simulink model "KTB1_SMAH"  (R2020a)
settings: Solver=ode45  StartTime=0.0  StopTime=120  RelTol=1e-3
values from neighbouring files (symbols this model uses):
  max_X = 5100    [SAP.m]
  max_XX = 2    [SAP.m]
  max_XXX = 0.05    [SAP.m]
  max_XXXX = 1050    [SAP.m]
  max_XXXXX = 15    [SAP.m]
  min_X = 0    [SAP.m]
  min_XX = 0    [SAP.m]
  min_XXX = 0    [SAP.m]
  min_XXXX = 0    [SAP.m]
  min_XXXXX = 0    [SAP.m]
  noiseseed = use2ndFcn    (= 1)    [SAP.m]
  noiseseed_X = use2ndFcn_X    (= 1)    [SAP.m]
  noiseseed_XX = use2ndFcn_XX    (= 1)    [SAP.m]
  noiseseed_XXX = use2ndFcn_XXX    (= 1)    [SAP.m]
  noiseseed_XXXX = use2ndFcn_XXXX    (= 1)    [SAP.m]
  noiseseed_XXXXX = use2ndFcn_XXXXX    (= 1)    [SAP.m]
  std = 0.025    [SAP.m]
  std_X = 0.025    [SAP.m]
  std_XX = 0.025    [SAP.m]
  std_XXX = 0.025    [SAP.m]
  std_XXXX = 0.025    [SAP.m]
  std_XXXXX = 0.025    [SAP.m]
  T_2 = T90_2/(24*60)/3.89    (= 0.000892602113682)    [SAP.m]
  T_8 = T90_8/(24*60)/11.7724    (= 0.00117978397683)    [SAP.m]
  T_X_2 = T90_X_2/(24*60)/3.89    (= 0.000892602113682)    [SAP.m]
  T_X_8 = T90_X_8/(24*60)/11.7724    (= 0.00117978397683)    [SAP.m]
  T_XX_2 = T90_XX_2/(24*60)/3.89    (= 0.000892602113682)    [SAP.m]
  T_XX_8 = T90_XX_8/(24*60)/11.7724    (= 0.00117978397683)    [SAP.m]
  T_XXX_2 = T90_XXX_2/(24*60)/3.89    (= 0.000892602113682)    [SAP.m]
  T_XXXX_2 = T90_XXXX_2/(24*60)/3.89    (= 0.000892602113682)    [SAP.m]
  T_XXXXX_2 = T90_XXXXX_2/(24*60)/3.89    (= 0.000892602113682)    [SAP.m]
  use2ndFcn = 1    [SAP.m]
  use2ndFcn_X = 1    [SAP.m]
  use2ndFcn_XX = 1    [SAP.m]
  use2ndFcn_XXX = 1    [SAP.m]
  use2ndFcn_XXXX = 1    [SAP.m]
  use2ndFcn_XXXXX = 1    [SAP.m]
  useideal = 1    [SAP.m]
  useideal_X = 1    [SAP.m]
  useideal_XX = 1    [SAP.m]
  useideal_XXX = 1    [SAP.m]
  useideal_XXXX = 1    [SAP.m]
  useideal_XXXXX = 1    [SAP.m]
  useidealac = 1    [SAP.m]
  useidealac_X = 1    [SAP.m]
  useidealac_XX = 1    [SAP.m]
  useidealac_XXX = 1    [SAP.m]
  useidealac_XXXX = 1    [SAP.m]
  useidealac_XXXXX = 1    [SAP.m]
  usenoise = 0    [SAP.m]
  usenoise_X = 0    [SAP.m]
  usenoise_XX = 0    [SAP.m]
  usenoise_XXX = 0    [SAP.m]
  usenoise_XXXX = 0    [SAP.m]
  usenoise_XXXXX = 0    [SAP.m]
libraries: simulink x6
(part 1 of 2)
settings Model: Creator=s182032  LastModifiedBy=morebo
settings DataIOCC: ReturnWorkspaceOutputs=off
settings DebuggingCC: MaxConsecutiveZCsMsg=none  ArithmeticOperatorsInVariantConditions=warning
settings SFSimCC: SimUseLocalCustomCode=off  CustomCodeUndefinedFunction=UseInterfaceOnly
settings RTWCC: RTWUseLocalCustomCode=off

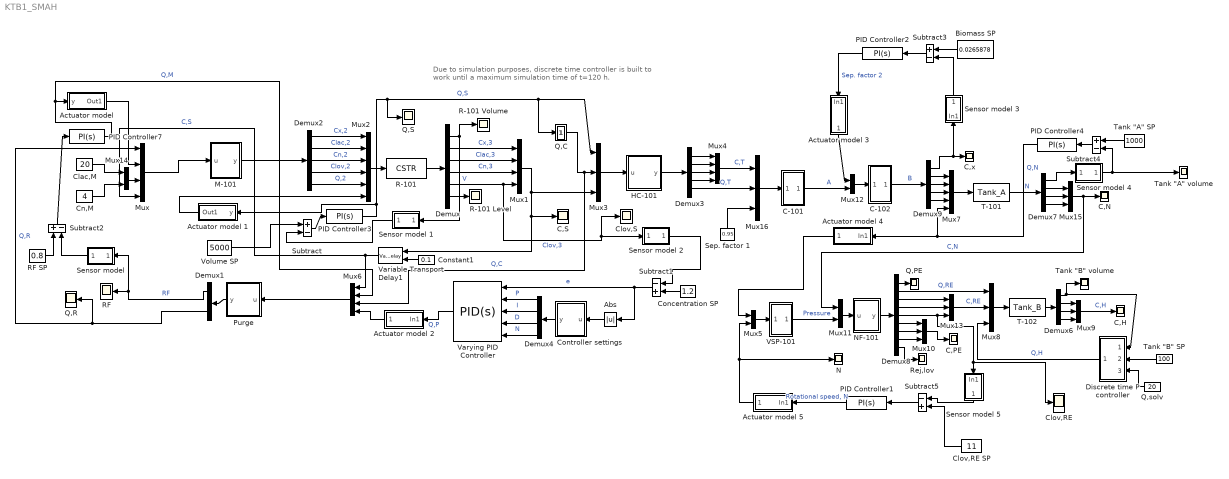
== system KTB1_SMAH ==
  note: Due to simulation purposes, discrete time controller is built to work until a maximum simulation time of t=120 h.
  Abs : Abs
  Actuator model : Subsystem
  Actuator model 1 : Subsystem
  Actuator model 2 : Subsystem
  Actuator model 3 : Subsystem
  Actuator model 4 : Subsystem
  Actuator model 5 : Subsystem
  Biomass SP : Constant  Value=0.0265878
  C,H : Scope
  C,N : Scope
  C,PE : Scope
  C,S : Scope
  C,x : Scope
  C-101 : MATLAB Function  TreatAsAtomicUnit=on
  C-102 : MATLAB Function  TreatAsAtomicUnit=on
  Clac,M : Constant  Value=20
  Clov,RE : Scope
  Clov,RE SP : Constant  Value=11
  Clov,S : Scope
  Cn,M : Constant  Value=4
  Concentration SP : Constant  Value=1.2
  Constant1 : Constant  Value=0.1
  Controller settings : MATLAB Function  TreatAsAtomicUnit=on
  Demux : Demux  Outputs=6
  Demux1 : Demux  Outputs=2
  Demux2 : Demux  Outputs=5
  Demux3 : Demux  Outputs=5
  Demux4 : Demux
  Demux6 : Demux
  Demux7 : Demux
  Demux8 : Demux  Outputs=9
  Demux9 : Demux  Outputs=5
  Discrete time P controller : Subsystem
  HC-101 : MATLAB Function  TreatAsAtomicUnit=on
  M-101 : MATLAB Function  TreatAsAtomicUnit=on
  Mux{,1,4,6} (4 alike) : Mux
  Mux{3,8..10,13,15..16} (7 alike) : Mux  Inputs=3
  Mux{5,11..12,14} (4 alike) : Mux  Inputs=2
  Mux2 : Mux  Inputs=6
  Mux7 : Mux  Inputs=5
  N : Scope
  NF-101 : MATLAB Function  TreatAsAtomicUnit=on
  PID Controller1 : simulink/Continuous/PID Controller  Controller=PI  Form=Parallel  TimeDomain=Continuous-time  UseExternalTs=off  SampleTime=-1  IntegratorMethod=Forward Euler  FilterMethod=Forward Euler  ControllerParametersSource=internal  P=0.234567821807165  I=0.999999996666666*0.234567821807165  D=0  UseFilter=on  N=100  TunerSelectOption=Transfer Function Based (PID Tuner App)  InitialConditionSource=internal  InitialConditionForIntegrator=3000  InitialConditionForFilter=0  DifferentiatorICPrevScaledInput=0  ExternalReset=none  TrackingMode=off  Kt=1  LimitOutput=on  UpperSaturationLimit=inf  LowerSaturationLimit=0  LinearizeAsGain=on  AntiWindupMode=clamping  Kb=1  POutMin=[]  POutMax=[]  IOutMin=[]  IOutMax=[]  DOutMin=[]  DOutMax=[]  NOutMin=[]  NOutMax=[]  SumOutMin=[]  SumOutMax=[]  SaturationOutMin=[]  SaturationOutMax=[]  PParamMin=[]  PParamMax=[]  IParamMin=[]  IParamMax=[]  DParamMin=[]  DParamMax=[]  NParamMin=[]  NParamMax=[]  KbParamMin=[]  KbParamMax=[]  KtParamMin=[]  KtParamMax=[]  KbOutMin=[]  KbOutMax=[]  KtOutMin=[]  KtOutMax=[]  IntegratorOutMin=[]  IntegratorOutMax=[]  FilterOutMin=[]  FilterOutMax=[]  SumI1OutMin=[]  SumI1OutMax=[]  SumI2OutMin=[]  SumI2OutMax=[]  SumI3OutMin=[]  SumI3OutMax=[]  SumI4OutMin=[]  SumI4OutMax=[]  SumDOutMin=[]  SumDOutMax=[]  DifferentiatorOutMin=[]  DifferentiatorOutMax=[]  FilterDiffOutCoefMin=[]  FilterDiffOutCoefMax=[]  ReciprocalOutMin=[]  ReciprocalOutMax=[]  SumDenOutMin=[]  SumDenOutMax=[]  SumNumOutMin=[]  SumNumOutMax=[]  DivideOutMin=[]  DivideOutMax=[]  UdiffTsProdOutMin=[]  UdiffTsProdOutMax=[]  NTsProdOutMin=[]  NTsProdOutMax=[]  UintegralTsProdOutMin=[]  UintegralTsProdOutMax=[]  UngainTsProdOutMin=[]  UngainTsProdOutMax=[]  IntegratorContinuousStateAttributes=''  IntegratorStateMustResolveToSignalObject=off  IntegratorRTWStateStorageClass=Auto  FilterContinuousStateAttributes=''  FilterStateMustResolveToSignalObject=off  FilterRTWStateStorageClass=Auto  ParallelPVariant=InternalParameters  IdealPVariant=Disabled  IVariant=InternalParameters  DVariant=Disabled  IntegratorVariant=Continuous  SatVariant=Enabled  AWVariant=ContClampingParallel  PCopyVariant=Disabled  TRVariant=Disabled  FdbkBlocksVariant=Forward  IdealPFdbkVariant=Disabled  SatFdbkVariant=Disabled  DerivativeFilterVariant=Disabled  NVariant=Disabled  NCopyVariant=Disabled_SignalSpec  FilterICVariant=Disabled  IntegratorICVariant=InternalICs  ExternalResetVariant=Disabled  TRSumVariant=Passthrough  SumFdbkVariant=Disabled  SumVariant=Sum_PI  TsampFilterVariant=InternalTs  TsampNgainVariant=Passthrough  TsampIntegralVariant=Passthrough
  PID Controller2 : simulink/Continuous/PID Controller  Controller=PI  Form=Parallel  TimeDomain=Continuous-time  UseExternalTs=off  SampleTime=-1  IntegratorMethod=Forward Euler  FilterMethod=Forward Euler  ControllerParametersSource=internal  P=-0.000476190628986061  I=9.99999996666667*(-0.000476190628986061)  D=0  UseFilter=on  N=100  TunerSelectOption=Transfer Function Based (PID Tuner App)  InitialConditionSource=internal  InitialConditionForIntegrator=0.95  InitialConditionForFilter=0  DifferentiatorICPrevScaledInput=0  ExternalReset=none  TrackingMode=off  Kt=1  LimitOutput=on  UpperSaturationLimit=0.98  LowerSaturationLimit=0  LinearizeAsGain=on  AntiWindupMode=clamping  Kb=1  POutMin=[]  POutMax=[]  IOutMin=[]  IOutMax=[]  DOutMin=[]  DOutMax=[]  NOutMin=[]  NOutMax=[]  SumOutMin=[]  SumOutMax=[]  SaturationOutMin=[]  SaturationOutMax=[]  PParamMin=[]  PParamMax=[]  IParamMin=[]  IParamMax=[]  DParamMin=[]  DParamMax=[]  NParamMin=[]  NParamMax=[]  KbParamMin=[]  KbParamMax=[]  KtParamMin=[]  KtParamMax=[]  KbOutMin=[]  KbOutMax=[]  KtOutMin=[]  KtOutMax=[]  IntegratorOutMin=[]  IntegratorOutMax=[]  FilterOutMin=[]  FilterOutMax=[]  SumI1OutMin=[]  SumI1OutMax=[]  SumI2OutMin=[]  SumI2OutMax=[]  SumI3OutMin=[]  SumI3OutMax=[]  SumI4OutMin=[]  SumI4OutMax=[]  SumDOutMin=[]  SumDOutMax=[]  DifferentiatorOutMin=[]  DifferentiatorOutMax=[]  FilterDiffOutCoefMin=[]  FilterDiffOutCoefMax=[]  ReciprocalOutMin=[]  ReciprocalOutMax=[]  SumDenOutMin=[]  SumDenOutMax=[]  SumNumOutMin=[]  SumNumOutMax=[]  DivideOutMin=[]  DivideOutMax=[]  UdiffTsProdOutMin=[]  UdiffTsProdOutMax=[]  NTsProdOutMin=[]  NTsProdOutMax=[]  UintegralTsProdOutMin=[]  UintegralTsProdOutMax=[]  UngainTsProdOutMin=[]  UngainTsProdOutMax=[]  IntegratorContinuousStateAttributes=''  IntegratorStateMustResolveToSignalObject=off  IntegratorRTWStateStorageClass=Auto  FilterContinuousStateAttributes=''  FilterStateMustResolveToSignalObject=off  FilterRTWStateStorageClass=Auto  ParallelPVariant=InternalParameters  IdealPVariant=Disabled  IVariant=InternalParameters  DVariant=Disabled  IntegratorVariant=Continuous  SatVariant=Enabled  AWVariant=ContClampingParallel  PCopyVariant=Disabled  TRVariant=Disabled  FdbkBlocksVariant=Forward  IdealPFdbkVariant=Disabled  SatFdbkVariant=Disabled  DerivativeFilterVariant=Disabled  NVariant=Disabled  NCopyVariant=Disabled_SignalSpec  FilterICVariant=Disabled  IntegratorICVariant=InternalICs  ExternalResetVariant=Disabled  TRSumVariant=Passthrough  SumFdbkVariant=Disabled  SumVariant=Sum_PI  TsampFilterVariant=InternalTs  TsampNgainVariant=Passthrough  TsampIntegralVariant=Passthrough
  PID Controller3 : simulink/Continuous/PID Controller  Controller=PI  Form=Parallel  TimeDomain=Continuous-time  UseExternalTs=off  SampleTime=-1  IntegratorMethod=Forward Euler  FilterMethod=Forward Euler  ControllerParametersSource=internal  P=-1/0.4/0.2  I=-1/0.4/0.2/4/0.2  D=0  UseFilter=on  N=100  TunerSelectOption=Transfer Function Based (PID Tuner App)  InitialConditionSource=internal  InitialConditionForIntegrator=64.0830509473650  InitialConditionForFilter=0  DifferentiatorICPrevScaledInput=0  ExternalReset=none  TrackingMode=off  Kt=1  LimitOutput=on  UpperSaturationLimit=inf  LowerSaturationLimit=0  LinearizeAsGain=on  AntiWindupMode=clamping  Kb=1  POutMin=[]  POutMax=[]  IOutMin=[]  IOutMax=[]  DOutMin=[]  DOutMax=[]  NOutMin=[]  NOutMax=[]  SumOutMin=[]  SumOutMax=[]  SaturationOutMin=[]  SaturationOutMax=[]  PParamMin=[]  PParamMax=[]  IParamMin=[]  IParamMax=[]  DParamMin=[]  DParamMax=[]  NParamMin=[]  NParamMax=[]  KbParamMin=[]  KbParamMax=[]  KtParamMin=[]  KtParamMax=[]  KbOutMin=[]  KbOutMax=[]  KtOutMin=[]  KtOutMax=[]  IntegratorOutMin=[]  IntegratorOutMax=[]  FilterOutMin=[]  FilterOutMax=[]  SumI1OutMin=[]  SumI1OutMax=[]  SumI2OutMin=[]  SumI2OutMax=[]  SumI3OutMin=[]  SumI3OutMax=[]  SumI4OutMin=[]  SumI4OutMax=[]  SumDOutMin=[]  SumDOutMax=[]  DifferentiatorOutMin=[]  DifferentiatorOutMax=[]  FilterDiffOutCoefMin=[]  FilterDiffOutCoefMax=[]  ReciprocalOutMin=[]  ReciprocalOutMax=[]  SumDenOutMin=[]  SumDenOutMax=[]  SumNumOutMin=[]  SumNumOutMax=[]  DivideOutMin=[]  DivideOutMax=[]  UdiffTsProdOutMin=[]  UdiffTsProdOutMax=[]  NTsProdOutMin=[]  NTsProdOutMax=[]  UintegralTsProdOutMin=[]  UintegralTsProdOutMax=[]  UngainTsProdOutMin=[]  UngainTsProdOutMax=[]  IntegratorContinuousStateAttributes=''  IntegratorStateMustResolveToSignalObject=off  IntegratorRTWStateStorageClass=Auto  FilterContinuousStateAttributes=''  FilterStateMustResolveToSignalObject=off  FilterRTWStateStorageClass=Auto  ParallelPVariant=InternalParameters  IdealPVariant=Disabled  IVariant=InternalParameters  DVariant=Disabled  IntegratorVariant=Continuous  SatVariant=Enabled  AWVariant=ContClampingParallel  PCopyVariant=Disabled  TRVariant=Disabled  FdbkBlocksVariant=Forward  IdealPFdbkVariant=Disabled  SatFdbkVariant=Disabled  DerivativeFilterVariant=Disabled  NVariant=Disabled  NCopyVariant=Disabled_SignalSpec  FilterICVariant=Disabled  IntegratorICVariant=InternalICs  ExternalResetVariant=Disabled  TRSumVariant=Passthrough  SumFdbkVariant=Disabled  SumVariant=Sum_PI  TsampFilterVariant=InternalTs  TsampNgainVariant=Passthrough  TsampIntegralVariant=Passthrough
  PID Controller4 : simulink/Continuous/PID Controller  Controller=PI  Form=Parallel  TimeDomain=Continuous-time  UseExternalTs=off  SampleTime=-1  IntegratorMethod=Forward Euler  FilterMethod=Forward Euler  ControllerParametersSource=internal  P=-1/140  I=-1/4/140/140  D=0  UseFilter=on  N=100  TunerSelectOption=Transfer Function Based (PID Tuner App)  InitialConditionSource=internal  InitialConditionForIntegrator=25.6332203789471  InitialConditionForFilter=0  DifferentiatorICPrevScaledInput=0  ExternalReset=none  TrackingMode=off  Kt=1  LimitOutput=on  UpperSaturationLimit=inf  LowerSaturationLimit=0  LinearizeAsGain=on  AntiWindupMode=clamping  Kb=1  POutMin=[]  POutMax=[]  IOutMin=[]  IOutMax=[]  DOutMin=[]  DOutMax=[]  NOutMin=[]  NOutMax=[]  SumOutMin=[]  SumOutMax=[]  SaturationOutMin=[]  SaturationOutMax=[]  PParamMin=[]  PParamMax=[]  IParamMin=[]  IParamMax=[]  DParamMin=[]  DParamMax=[]  NParamMin=[]  NParamMax=[]  KbParamMin=[]  KbParamMax=[]  KtParamMin=[]  KtParamMax=[]  KbOutMin=[]  KbOutMax=[]  KtOutMin=[]  KtOutMax=[]  IntegratorOutMin=[]  IntegratorOutMax=[]  FilterOutMin=[]  FilterOutMax=[]  SumI1OutMin=[]  SumI1OutMax=[]  SumI2OutMin=[]  SumI2OutMax=[]  SumI3OutMin=[]  SumI3OutMax=[]  SumI4OutMin=[]  SumI4OutMax=[]  SumDOutMin=[]  SumDOutMax=[]  DifferentiatorOutMin=[]  DifferentiatorOutMax=[]  FilterDiffOutCoefMin=[]  FilterDiffOutCoefMax=[]  ReciprocalOutMin=[]  ReciprocalOutMax=[]  SumDenOutMin=[]  SumDenOutMax=[]  SumNumOutMin=[]  SumNumOutMax=[]  DivideOutMin=[]  DivideOutMax=[]  UdiffTsProdOutMin=[]  UdiffTsProdOutMax=[]  NTsProdOutMin=[]  NTsProdOutMax=[]  UintegralTsProdOutMin=[]  UintegralTsProdOutMax=[]  UngainTsProdOutMin=[]  UngainTsProdOutMax=[]  IntegratorContinuousStateAttributes=''  IntegratorStateMustResolveToSignalObject=off  IntegratorRTWStateStorageClass=Auto  FilterContinuousStateAttributes=''  FilterStateMustResolveToSignalObject=off  FilterRTWStateStorageClass=Auto  ParallelPVariant=InternalParameters  IdealPVariant=Disabled  IVariant=InternalParameters  DVariant=Disabled  IntegratorVariant=Continuous  SatVariant=Enabled  AWVariant=ContClampingParallel  PCopyVariant=Disabled  TRVariant=Disabled  FdbkBlocksVariant=Forward  IdealPFdbkVariant=Disabled  SatFdbkVariant=Disabled  DerivativeFilterVariant=Disabled  NVariant=Disabled  NCopyVariant=Disabled_SignalSpec  FilterICVariant=Disabled  IntegratorICVariant=InternalICs  ExternalResetVariant=Disabled  TRSumVariant=Passthrough  SumFdbkVariant=Disabled  SumVariant=Sum_PI  TsampFilterVariant=InternalTs  TsampNgainVariant=Passthrough  TsampIntegralVariant=Passthrough
  PID Controller7 : simulink/Continuous/PID Controller  Controller=PI  Form=Parallel  TimeDomain=Continuous-time  UseExternalTs=off  SampleTime=-1  IntegratorMethod=Forward Euler  FilterMethod=Forward Euler  ControllerParametersSource=internal  P=4.68116891262785/100  I=30.3539293345611/100  D=0  UseFilter=on  N=100  TunerSelectOption=Transfer Function Based (PID Tuner App)  InitialConditionSource=internal  InitialConditionForIntegrator=35.6016949707568  InitialConditionForFilter=0  DifferentiatorICPrevScaledInput=0  ExternalReset=none  TrackingMode=off  Kt=1  LimitOutput=on  UpperSaturationLimit=inf  LowerSaturationLimit=0  LinearizeAsGain=on  AntiWindupMode=clamping  Kb=1  POutMin=[]  POutMax=[]  IOutMin=[]  IOutMax=[]  DOutMin=[]  DOutMax=[]  NOutMin=[]  NOutMax=[]  SumOutMin=[]  SumOutMax=[]  SaturationOutMin=[]  SaturationOutMax=[]  PParamMin=[]  PParamMax=[]  IParamMin=[]  IParamMax=[]  DParamMin=[]  DParamMax=[]  NParamMin=[]  NParamMax=[]  KbParamMin=[]  KbParamMax=[]  KtParamMin=[]  KtParamMax=[]  KbOutMin=[]  KbOutMax=[]  KtOutMin=[]  KtOutMax=[]  IntegratorOutMin=[]  IntegratorOutMax=[]  FilterOutMin=[]  FilterOutMax=[]  SumI1OutMin=[]  SumI1OutMax=[]  SumI2OutMin=[]  SumI2OutMax=[]  SumI3OutMin=[]  SumI3OutMax=[]  SumI4OutMin=[]  SumI4OutMax=[]  SumDOutMin=[]  SumDOutMax=[]  DifferentiatorOutMin=[]  DifferentiatorOutMax=[]  FilterDiffOutCoefMin=[]  FilterDiffOutCoefMax=[]  ReciprocalOutMin=[]  ReciprocalOutMax=[]  SumDenOutMin=[]  SumDenOutMax=[]  SumNumOutMin=[]  SumNumOutMax=[]  DivideOutMin=[]  DivideOutMax=[]  UdiffTsProdOutMin=[]  UdiffTsProdOutMax=[]  NTsProdOutMin=[]  NTsProdOutMax=[]  UintegralTsProdOutMin=[]  UintegralTsProdOutMax=[]  UngainTsProdOutMin=[]  UngainTsProdOutMax=[]  IntegratorContinuousStateAttributes=''  IntegratorStateMustResolveToSignalObject=off  IntegratorRTWStateStorageClass=Auto  FilterContinuousStateAttributes=''  FilterStateMustResolveToSignalObject=off  FilterRTWStateStorageClass=Auto  ParallelPVariant=InternalParameters  IdealPVariant=Disabled  IVariant=InternalParameters  DVariant=Disabled  IntegratorVariant=Continuous  SatVariant=Enabled  AWVariant=ContClampingParallel  PCopyVariant=Disabled  TRVariant=Disabled  FdbkBlocksVariant=Forward  IdealPFdbkVariant=Disabled  SatFdbkVariant=Disabled  DerivativeFilterVariant=Disabled  NVariant=Disabled  NCopyVariant=Disabled_SignalSpec  FilterICVariant=Disabled  IntegratorICVariant=InternalICs  ExternalResetVariant=Disabled  TRSumVariant=Passthrough  SumFdbkVariant=Disabled  SumVariant=Sum_PI  TsampFilterVariant=InternalTs  TsampNgainVariant=Passthrough  TsampIntegralVariant=Passthrough
  Purge : MATLAB Function  TreatAsAtomicUnit=on
  Q,C : Subsystem
  Q,PE : Scope
  Q,R : Scope
  Q,S : Scope
  Q,solv : Constant  Value=20
  R-101 : S-Function  FunctionName=CSTR  SFunctionDeploymentMode=off  EnableBusSupport=off
  R-101 Level : Scope
  R-101 Volume : Scope
  RF : Scope
  RF SP : Constant  Value=0.8
  Rej,lov : Scope
  Sensor model : Subsystem
  Sensor model 1 : Subsystem
  Sensor model 2 : Subsystem
  Sensor model 3 : Subsystem
  Sensor model 4 : Subsystem
  Sensor model 5 : Subsystem
  Sep. factor 1 : Constant  Value=0.95
  Subtract{,2..4} (4 alike) : Sum  Inputs=+-
  Subtract1 : Sum  Inputs=-+
  Subtract5 : Sum  Inputs=-+
  T-101 : S-Function  FunctionName=Tank_A  SFunctionDeploymentMode=off  EnableBusSupport=off
  T-102 : S-Function  FunctionName=Tank_B  SFunctionDeploymentMode=off  EnableBusSupport=off
  "Tank \"A\" SP" : Constant  Value=1000
  "Tank \"A\" volume" : Scope
  "Tank \"B\" SP" : Constant  Value=100
  "Tank \"B\" volume" : Scope
  VSP-101 : MATLAB Function  TreatAsAtomicUnit=on
  Variable Transport Delay1 : VariableTransportDelay  VariableDelayType=Variable transport delay  MaximumDelay=10  InitialOutput=[106.351163614666 14.8096563646109 2.51553709810012 1.20000000000003]  MaximumPoints=80000
  Varying PID Controller : simulink/Continuous/PID Controller  Controller=PID  Form=Parallel  TimeDomain=Continuous-time  UseExternalTs=off  SampleTime=-1  IntegratorMethod=Forward Euler  FilterMethod=Forward Euler  ControllerParametersSource=external  P=1  I=1  D=0  UseFilter=on  N=100  TunerSelectOption=Transfer Function Based (PID Tuner App)  InitialConditionSource=internal  InitialConditionForIntegrator=9.96847459181301  InitialConditionForFilter=0  DifferentiatorICPrevScaledInput=0  ExternalReset=none  TrackingMode=off  Kt=1  LimitOutput=on  UpperSaturationLimit=inf  LowerSaturationLimit=0  LinearizeAsGain=on  AntiWindupMode=none  Kb=1  POutMin=[]  POutMax=[]  IOutMin=[]  IOutMax=[]  DOutMin=[]  DOutMax=[]  NOutMin=[]  NOutMax=[]  SumOutMin=[]  SumOutMax=[]  SaturationOutMin=[]  SaturationOutMax=[]  PParamMin=[]  PParamMax=[]  IParamMin=[]  IParamMax=[]  DParamMin=[]  DParamMax=[]  NParamMin=[]  NParamMax=[]  KbParamMin=[]  KbParamMax=[]  KtParamMin=[]  KtParamMax=[]  KbOutMin=[]  KbOutMax=[]  KtOutMin=[]  KtOutMax=[]  IntegratorOutMin=[]  IntegratorOutMax=[]  FilterOutMin=[]  FilterOutMax=[]  SumI1OutMin=[]  SumI1OutMax=[]  SumI2OutMin=[]  SumI2OutMax=[]  SumI3OutMin=[]  SumI3OutMax=[]  SumI4OutMin=[]  SumI4OutMax=[]  SumDOutMin=[]  SumDOutMax=[]  DifferentiatorOutMin=[]  DifferentiatorOutMax=[]  FilterDiffOutCoefMin=[]  FilterDiffOutCoefMax=[]  ReciprocalOutMin=[]  ReciprocalOutMax=[]  SumDenOutMin=[]  SumDenOutMax=[]  SumNumOutMin=[]  SumNumOutMax=[]  DivideOutMin=[]  DivideOutMax=[]  UdiffTsProdOutMin=[]  UdiffTsProdOutMax=[]  NTsProdOutMin=[]  NTsProdOutMax=[]  UintegralTsProdOutMin=[]  UintegralTsProdOutMax=[]  UngainTsProdOutMin=[]  UngainTsProdOutMax=[]  IntegratorContinuousStateAttributes=''  IntegratorStateMustResolveToSignalObject=off  IntegratorRTWStateStorageClass=Auto  FilterContinuousStateAttributes=''  FilterStateMustResolveToSignalObject=off  FilterRTWStateStorageClass=Auto  ParallelPVariant=ExternalParameters  IdealPVariant=Disabled  IVariant=ExternalParameters  DVariant=ExternalParameters  IntegratorVariant=Continuous  SatVariant=Enabled  AWVariant=Passthrough  PCopyVariant=Disabled  TRVariant=Disabled  FdbkBlocksVariant=Forward  IdealPFdbkVariant=Disabled  SatFdbkVariant=Disabled  DerivativeFilterVariant=ContFilter  NVariant=ExternalParameters  NCopyVariant=Disabled  FilterICVariant=InternalICsFilter  IntegratorICVariant=InternalICs  ExternalResetVariant=Disabled  TRSumVariant=Passthrough  SumFdbkVariant=Disabled  SumVariant=Sum_PID  TsampFilterVariant=InternalTs  TsampNgainVariant=Passthrough  TsampIntegralVariant=Passthrough
  Volume SP : Constant  Value=5000
  wires:
  Concentration SP/1 -> Subtract1/2
  Demux4/1 -> Varying PID Controller/2  "P"
  Subtract1/1 -> Abs/1, Varying PID Controller/1  "e"
  Demux4/2 -> Varying PID Controller/3  "I"
  PID Controller7/1 -> Actuator model/1(y), Mux6/2  "Q,M"
  Varying PID Controller/1 -> Actuator model 2/1(In1)  "Q,P"
  Demux2/5 -> Mux2/5  "Q,2"
  Mux6/1 -> Purge/1(u)
  Demux2/4 -> Mux2/4  "Clov,2"
  Demux3/1 -> Mux4/1
  Purge/1(y) -> Demux1/1
  Demux2/3 -> Mux2/3  "Cn,2"
  Demux3/2 -> Mux4/2
  Demux3/3 -> Mux4/3
  HC-101/1(y) -> Demux3/1
  Mux3/1 -> HC-101/1(u)
  Demux2/2 -> Mux2/2  "Clac,2"
  PID Controller3/1 -> Actuator model 1/1(y), Q,C/1(Qs), Mux3/1, Q,S/1  "Q,S"
  Demux/1 -> Sensor model 1/1(In1), R-101 Volume/1  "V"
  Demux/2 -> Mux1/1  "Cx,3"
  Demux/3 -> Mux1/2  "Clac,3"
  Mux/1 -> M-101/1(u)
  Mux2/1 -> R-101/1
  Demux2/1 -> Mux2/1  "Cx,2"
  Variable Transport Delay1/1 -> Mux/4, Mux6/1  "C,S"
  R-101/1 -> Demux/1
  Mux1/1 -> C,S/1, Variable Transport Delay1/1, Mux3/3
  Constant1/1 -> Variable Transport Delay1/2
  M-101/1(y) -> Demux2/1
  Demux/4 -> Mux1/3  "Cn,3"
  Demux/5 -> Clov,S/1, Sensor model 2/1(In1), Mux1/4  "Clov,3"
  Subtract/1 -> PID Controller3/1
  Demux3/4 -> Mux4/4
  Cn,M/1 -> Mux14/2
  Demux/6 -> R-101 Level/1
  Mux14/1 -> Mux/3
  Demux1/2 -> Mux/1, Q,R/1  "Q,R"
  Volume SP/1 -> Subtract/1
  Demux1/1 -> Sensor model/1(In1), RF/1  "RF"
  Clac,M/1 -> Mux14/1
  Abs/1 -> Controller settings/1(u)
  Controller settings/1(y) -> Demux4/1
  Demux4/3 -> Varying PID Controller/4  "D"
  Demux4/4 -> Varying PID Controller/5  "N"
  RF SP/1 -> Subtract2/1
  Subtract2/1 -> PID Controller7/1
  Q,C/1(Qc) -> Mux6/3, Mux3/2  "Q,C"
  Demux6/1 -> Discrete time P controller/1(In1), "Tank \"B\" volume"/1
  Discrete time P controller/1(Q,H) -> Mux8/3  "Q,H"
  Q,solv/1 -> Discrete time P controller/3(In3)
  "Tank \"B\" SP"/1 -> Discrete time P controller/2(In2)
  Demux9/4 -> Mux7/3
  Clov,RE SP/1 -> Subtract5/2
  Subtract3/1 -> PID Controller2/1
  C-102/1(y) -> Demux9/1  "B"
  Demux8/9 -> Rej,lov/1
  PID Controller1/1 -> Actuator model 5/1(In1)  "Rotational speed, N"
  Demux9/1 -> Sensor model 3/1(In1), C,x/1
  Demux7/3 -> Mux15/2
  Demux8/8 -> Mux10/3
  Demux9/2 -> Mux7/1
  Mux5/1 -> VSP-101/1(u)
  VSP-101/1(y) -> Mux11/2  "Pressure"
  Demux6/2 -> Mux9/1
  T-102/1 -> Demux6/1
  Demux9/5 -> Mux7/4
  Demux8/2 -> Mux8/1  "Q,RE"
  Demux6/3 -> Mux9/2
  Mux15/1 -> Mux11/1, C,N/1  "C,N"
  Mux7/1 -> T-101/1
  Demux9/3 -> Mux7/2
  Demux8/3 -> Mux13/1
  Mux8/1 -> T-102/1
  Mux10/1 -> C,PE/1
  Demux8/4 -> Mux13/2
  Subtract4/1 -> PID Controller4/1
  PID Controller4/1 -> Actuator model 4/1(In1), Mux7/5  "Q,N"
  Subtract5/1 -> PID Controller1/1
  Demux8/7 -> Mux10/2
  Demux6/4 -> Mux9/3
  Mux16/1 -> C-101/1(u)
  Sep. factor 1/1 -> Mux16/3
  Mux11/1 -> NF-101/1(u)
  NF-101/1(y) -> Demux8/1
  "Tank \"A\" SP"/1 -> Subtract4/1
  Mux9/1 -> C,H/1  "C,H"
  T-101/1 -> Demux7/1  "N"
  Mux13/1 -> Mux8/2  "C,RE"
  Mux12/1 -> C-102/1(u)
  Biomass SP/1 -> Subtract3/1
  Demux8/6 -> Mux10/1
  Demux7/4 -> Mux15/3
  Demux8/1 -> Q,PE/1
  C-101/1(y) -> Mux12/2  "A"
  Demux7/2 -> Mux15/1
  PID Controller2/1 -> Actuator model 3/1(In1)  "Sep. factor 2"
  Mux4/1 -> Mux16/1  "C,T"
  Demux3/5 -> Mux16/2  "Q,T"
  Sensor model 2/1(Out1) -> Subtract1/1
  Actuator model 2/1(Out1) -> Mux6/4
  Sensor model/1(Out1) -> Subtract2/2
  Actuator model/1(Out1) -> Mux/2
  Sensor model 1/1(Out1) -> Subtract/2
  Actuator model 1/1(Out1) -> Mux2/6
  Sensor model 3/1(Out1) -> Subtract3/2
  Actuator model 3/1(Out1) -> Mux12/1
  Demux7/1 -> Sensor model 4/1(In1)
  Demux8/5 -> Clov,RE/1, Sensor model 5/1(In1), Mux13/3
  Sensor model 4/1(Out1) -> Subtract4/2, "Tank \"A\" volume"/1
  Actuator model 4/1(Out1) -> Mux5/1
  Sensor model 5/1(Out1) -> Subtract5/1
  Actuator model 5/1(Out1) -> Mux5/2, N/1

== system KTB1_SMAH/Actuator model ==
  y : Inport
  Constant2 : Constant  Value=useidealac
  Switch1 : Switch  Threshold=0.5
  actuator : TransferFcn  Denominator=[ T_2*T_2, 2*T_2, 1]
  Out1 : Outport
  wires:
  Constant2/1 -> Switch1/2
  y/1 -> Switch1/1, actuator/1
  actuator/1 -> Switch1/3
  Switch1/1 -> Out1/1

== system KTB1_SMAH/Actuator model 1 ==
  y : Inport
  Constant2 : Constant  Value=useidealac_X
  Switch1 : Switch  Threshold=0.5
  X_actuator : TransferFcn  Denominator=[ T_X_2*T_X_2, 2*T_X_2, 1]
  Out1 : Outport
  wires:
  Constant2/1 -> Switch1/2
  y/1 -> Switch1/1, X_actuator/1
  X_actuator/1 -> Switch1/3
  Switch1/1 -> Out1/1

== system KTB1_SMAH/Actuator model 2 ==
  In1 : Inport
  Constant2 : Constant  Value=useidealac_XX
  Switch1 : Switch  Threshold=0.5
  XX_actuator : TransferFcn  Denominator=[ T_XX_2*T_XX_2, 2*T_XX_2, 1]
  Out1 : Outport
  wires:
  Constant2/1 -> Switch1/2
  In1/1 -> Switch1/1, XX_actuator/1
  XX_actuator/1 -> Switch1/3
  Switch1/1 -> Out1/1

== system KTB1_SMAH/Actuator model 3 ==
  In1 : Inport
  Constant2 : Constant  Value=useidealac_XXX
  Switch1 : Switch  Threshold=0.5
  XXX_actuator : TransferFcn  Denominator=[ T_XXX_2*T_XXX_2, 2*T_XXX_2, 1]
  Out1 : Outport
  wires:
  Constant2/1 -> Switch1/2
  In1/1 -> Switch1/1, XXX_actuator/1
  XXX_actuator/1 -> Switch1/3
  Switch1/1 -> Out1/1

== system KTB1_SMAH/Actuator model 4 ==
  In1 : Inport
  Constant2 : Constant  Value=useidealac_XXXX
  Switch1 : Switch  Threshold=0.5
  XXXX_actuator : TransferFcn  Denominator=[ T_XXXX_2*T_XXXX_2, 2*T_XXXX_2, 1]
  Out1 : Outport
  wires:
  Constant2/1 -> Switch1/2
  In1/1 -> Switch1/1, XXXX_actuator/1
  XXXX_actuator/1 -> Switch1/3
  Switch1/1 -> Out1/1

== system KTB1_SMAH/Actuator model 5 ==
  In1 : Inport
  Constant2 : Constant  Value=useidealac_XXXXX
  Switch1 : Switch  Threshold=0.5
  XXXX_actuator : TransferFcn  Denominator=[ T_XXXXX_2*T_XXXXX_2, 2*T_XXXXX_2, 1]
  Out1 : Outport
  wires:
  Constant2/1 -> Switch1/2
  In1/1 -> Switch1/1, XXXX_actuator/1
  XXXX_actuator/1 -> Switch1/3
  Switch1/1 -> Out1/1

== system KTB1_SMAH/Discrete time P controller ==
  In1 : Inport
  In2 : Inport  Port=2
  In3 : Inport  Port=3
  1 : Subsystem
  10 : Subsystem
  2 : Subsystem
  3 : Subsystem
  4 : Subsystem
  5 : Subsystem
  6 : Subsystem
  7 : Subsystem
  8 : Subsystem
  9 : Subsystem
  Sum1 : Sum  Inputs=++++++++++
  Q,H : Outport  VectorParamsAs1DForOutWhenUnconnected=off
  wires:
  In3/1 -> 3/3(In3), 4/3(In3), 6/3(In3), 7/3(In3), 8/3(In3), 10/3(In3), 9/3(In3), 5/3(In3), 2/3(In3), 1/1(In1)
  In2/1 -> 2/2(In2), 3/2(In2), 4/2(In2), 5/2(In2), 6/2(In2), 8/2(In2), 10/2(In2), 9/2(In2), 7/2(In2)
  7/1(Out1) -> Sum1/7
  3/1(Out1) -> Sum1/3
  4/1(Out1) -> Sum1/4
  2/1(Out1) -> Sum1/2
  6/1(Out1) -> Sum1/6
  8/1(Out1) -> Sum1/8
  10/1(Out1) -> Sum1/10
  9/1(Out1) -> Sum1/9
  5/1(Out1) -> Sum1/5
  Sum1/1 -> Q,H/1  "Q,H"
  1/1(Out1) -> Sum1/1
  In1/1 -> 4/1(In1), 5/1(In1), 6/1(In1), 7/1(In1), 8/1(In1), 10/1(In1), 9/1(In1), 3/1(In1), 2/1(In1)

== system KTB1_SMAH/Q,C ==
  Qs : Inport
  Product1 : Product
  Q,C/Q,S : Constant  Value=0.6
  Qc : Outport  VectorParamsAs1DForOutWhenUnconnected=off
  wires:
  Product1/1 -> Qc/1  "Qc"
  Q,C/Q,S/1 -> Product1/1
  Qs/1 -> Product1/2

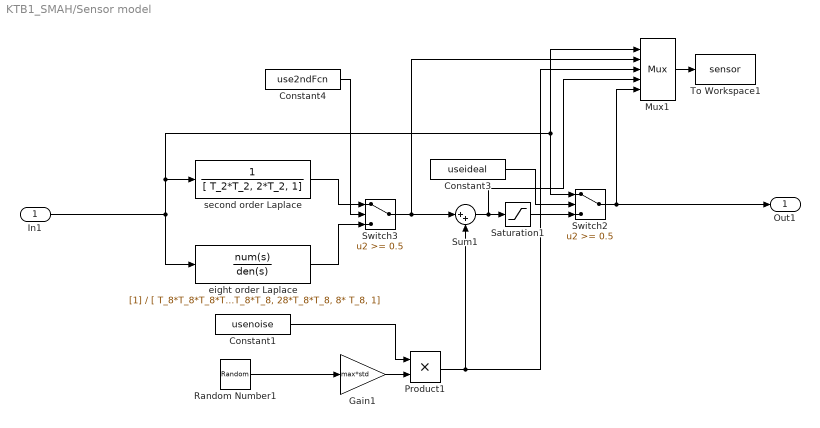
== system KTB1_SMAH/Sensor model ==
  In1 : Inport
  Constant1 : Constant  Value=usenoise
  Constant3 : Constant  Value=useideal
  Constant4 : Constant  Value=use2ndFcn
  Gain1 : Gain  Gain=max*std  SaturateOnIntegerOverflow=on  OutDataTypeStr=Inherit: Same as input  ParamDataTypeStr=Inherit: Same as input
  Mux1 : Mux  Inputs=5
  Product1 : Product  InputSameDT=on  SaturateOnIntegerOverflow=on  OutDataTypeStr=Inherit: Same as first input
  Random Number1 : RandomNumber  Seed=noiseseed  SampleTime=1/2
  Saturation1 : Saturate  UpperLimit=max  LowerLimit=min
  Sum1 : Sum  Inputs=|++  InputSameDT=on  SaturateOnIntegerOverflow=on  OutDataTypeStr=Inherit: Same as first input
  Switch2 : Switch  Threshold=0.5
  Switch3 : Switch  Threshold=0.5
  To Workspace1 : ToWorkspace  VariableName=sensor  SampleTime=-1
  eight order Laplace : TransferFcn  Denominator=[ T_8*T_8*T_8*T_8*T_8*T_8*T_8*T_8, 8*T_8*T_8*T_8*T_8*T_8*T_8*T_8, 28*T_8*T_8*T_8*T_8*T_8*T_8, 56*T_8*T_8*T_8*T_8*T_8, 70*T_8*T_8*T_8*T_8, 56*T_8*T_8*T_8, 28*T_8*T_8, 8* T_8, 1]
  second order Laplace : TransferFcn  Denominator=[ T_2*T_2, 2*T_2, 1]
  Out1 : Outport
  wires:
  Saturation1/1 -> Switch2/3
  In1/1 -> second order Laplace/1, Mux1/1, Switch2/1, eight order Laplace/1
  Constant1/1 -> Product1/1
  eight order Laplace/1 -> Switch3/3
  Constant4/1 -> Switch3/2
  Gain1/1 -> Product1/2
  Product1/1 -> Mux1/3, Sum1/2
  Switch2/1 -> Mux1/5, Out1/1
  Constant3/1 -> Switch2/2
  second order Laplace/1 -> Switch3/1
  Random Number1/1 -> Gain1/1
  Mux1/1 -> To Workspace1/1
  Sum1/1 -> Mux1/4, Saturation1/1
  Switch3/1 -> Mux1/2, Sum1/1

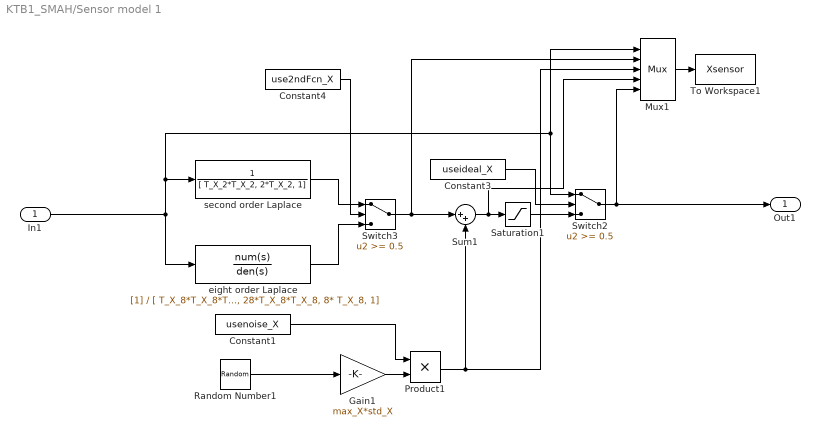
== system KTB1_SMAH/Sensor model 1 ==
  In1 : Inport
  Constant1 : Constant  Value=usenoise_X
  Constant3 : Constant  Value=useideal_X
  Constant4 : Constant  Value=use2ndFcn_X
  Gain1 : Gain  Gain=max_X*std_X  SaturateOnIntegerOverflow=on  OutDataTypeStr=Inherit: Same as input  ParamDataTypeStr=Inherit: Same as input
  Mux1 : Mux  Inputs=5
  Product1 : Product  InputSameDT=on  SaturateOnIntegerOverflow=on  OutDataTypeStr=Inherit: Same as first input
  Random Number1 : RandomNumber  Variance=0.0025  Seed=noiseseed_X  SampleTime=1/2
  Saturation1 : Saturate  UpperLimit=max_X  LowerLimit=min_X
  Sum1 : Sum  Inputs=|++  InputSameDT=on  SaturateOnIntegerOverflow=on  OutDataTypeStr=Inherit: Same as first input
  Switch2 : Switch  Threshold=0.5
  Switch3 : Switch  Threshold=0.5
  To Workspace1 : ToWorkspace  VariableName=Xsensor  SampleTime=-1
  eight order Laplace : TransferFcn  Denominator=[ T_X_8*T_X_8*T_X_8*T_X_8*T_X_8*T_X_8*T_X_8*T_X_8, 8*T_X_8*T_X_8*T_X_8*T_X_8*T_X_8*T_X_8*T_X_8, 28*T_X_8*T_X_8*T_X_8*T_X_8*T_X_8*T_X_8, 56*T_X_8*T_X_8*T_X_8*T_X_8*T_X_8, 70*T_X_8*T_X_8*T_X_8*T_X_8, 56*T_X_8*T_X_8*T_X_8, 28*T_X_8*T_X_8, 8* T_X_8, 1]
  second order Laplace : TransferFcn  Denominator=[ T_X_2*T_X_2, 2*T_X_2, 1]
  Out1 : Outport
  wires:
  Saturation1/1 -> Switch2/3
  In1/1 -> second order Laplace/1, Mux1/1, Switch2/1, eight order Laplace/1
  Constant1/1 -> Product1/1
  eight order Laplace/1 -> Switch3/3
  Constant4/1 -> Switch3/2
  Gain1/1 -> Product1/2
  Product1/1 -> Mux1/3, Sum1/2
  Switch2/1 -> Mux1/5, Out1/1
  Constant3/1 -> Switch2/2
  second order Laplace/1 -> Switch3/1
  Random Number1/1 -> Gain1/1
  Mux1/1 -> To Workspace1/1
  Sum1/1 -> Mux1/4, Saturation1/1
  Switch3/1 -> Mux1/2, Sum1/1

== system KTB1_SMAH/Sensor model 2 ==
  In1 : Inport
  Constant1 : Constant  Value=usenoise_XX
  Constant3 : Constant  Value=useideal_XX
  Constant4 : Constant  Value=use2ndFcn_XX
  Gain1 : Gain  Gain=max_XX*std_XX  SaturateOnIntegerOverflow=on  OutDataTypeStr=Inherit: Same as input  ParamDataTypeStr=Inherit: Same as input
  Mux1 : Mux  Inputs=5
  Product1 : Product  InputSameDT=on  SaturateOnIntegerOverflow=on  OutDataTypeStr=Inherit: Same as first input
  Random Number1 : RandomNumber  Variance=0.025  Seed=noiseseed_XX  SampleTime=1/2
  Saturation1 : Saturate  UpperLimit=max_XX  LowerLimit=min_XX
  Sum1 : Sum  Inputs=|++  InputSameDT=on  SaturateOnIntegerOverflow=on  OutDataTypeStr=Inherit: Same as first input
  Switch2 : Switch  Threshold=0.5
  Switch3 : Switch  Threshold=0.5
  To Workspace1 : ToWorkspace  VariableName=XXsensor  SampleTime=-1
  eight order Laplace : TransferFcn  Denominator=[ T_XX_8*T_XX_8*T_XX_8*T_XX_8*T_XX_8*T_XX_8*T_XX_8*T_XX_8, 8*T_XX_8*T_XX_8*T_XX_8*T_XX_8*T_XX_8*T_XX_8*T_XX_8, 28*T_XX_8*T_XX_8*T_XX_8*T_XX_8*T_XX_8*T_XX_8, 56*T_XX_8*T_XX_8*T_XX_8*T_XX_8*T_XX_8, 70*T_XX_8*T_XX_8*T_XX_8*T_XX_8, 56*T_XX_8*T_XX_8*T_XX_8, 28*T_XX_8*T_XX_8, 8* T_XX_8, 1]
  second order Laplace : TransferFcn  Denominator=[ T_XX_2*T_XX_2, 2*T_XX_2, 1]
  Out1 : Outport
  wires:
  Saturation1/1 -> Switch2/3
  In1/1 -> second order Laplace/1, Mux1/1, Switch2/1, eight order Laplace/1
  Constant1/1 -> Product1/1
  eight order Laplace/1 -> Switch3/3
  Constant4/1 -> Switch3/2
  Gain1/1 -> Product1/2
  Product1/1 -> Mux1/3, Sum1/2
  Switch2/1 -> Mux1/5, Out1/1
  Constant3/1 -> Switch2/2
  second order Laplace/1 -> Switch3/1
  Random Number1/1 -> Gain1/1
  Mux1/1 -> To Workspace1/1
  Sum1/1 -> Mux1/4, Saturation1/1
  Switch3/1 -> Mux1/2, Sum1/1

== system KTB1_SMAH/Sensor model 3 ==
  In1 : Inport
  Constant1 : Constant  Value=usenoise_XXX
  Constant3 : Constant  Value=useideal_XXX
  Constant4 : Constant  Value=use2ndFcn_XXX
  Gain1 : Gain  Gain=max_XXX*std_XXX  SaturateOnIntegerOverflow=on  OutDataTypeStr=Inherit: Same as input  ParamDataTypeStr=Inherit: Same as input
  Mux1 : Mux  Inputs=5
  Product1 : Product  InputSameDT=on  SaturateOnIntegerOverflow=on  OutDataTypeStr=Inherit: Same as first input
  Random Number1 : RandomNumber  Variance=0.025  Seed=noiseseed_XXX  SampleTime=1/2
  Saturation1 : Saturate  UpperLimit=max_XXX  LowerLimit=min_XXX
  Sum1 : Sum  Inputs=|++  InputSameDT=on  SaturateOnIntegerOverflow=on  OutDataTypeStr=Inherit: Same as first input
  Switch2 : Switch  Threshold=0.5
  Switch3 : Switch  Threshold=0.5
  To Workspace1 : ToWorkspace  VariableName=XXXsensor  SampleTime=-1
  eight order Laplace : TransferFcn  Denominator=[ T_XXX_8*T_XXX_8*T_XXX_8*T_XXX_8*T_XXX_8*T_XXX_8*T_XXX_8*T_XXX_8, 8*T_XXX_8*T_XXX_8*T_XXX_8*T_XXX_8*T_XXX_8*T_XXX_8*T_XXX_8, 28*T_XXX_8*T_XXX_8*T_XXX_8*T_XXX_8*T_XXX_8*T_XXX_8, 56*T_XXX_8*T_XXX_8*T_XXX_8*T_XXX_8*T_XXX_8, 70*T_XXX_8*T_XXX_8*T_XXX_8*T_XXX_8, 56*T_XXX_8*T_XXX_8*T_XXX_8, 28*T_XXX_8*T_XXX_8, 8* T_XXX_8, 1]
  second order Laplace : TransferFcn  Denominator=[ T_XXX_2*T_XXX_2, 2*T_XXX_2, 1]
  Out1 : Outport
  wires:
  Saturation1/1 -> Switch2/3
  In1/1 -> second order Laplace/1, Mux1/1, Switch2/1, eight order Laplace/1
  Constant1/1 -> Product1/1
  eight order Laplace/1 -> Switch3/3
  Constant4/1 -> Switch3/2
  Gain1/1 -> Product1/2
  Product1/1 -> Mux1/3, Sum1/2
  Switch2/1 -> Mux1/5, Out1/1
  Constant3/1 -> Switch2/2
  second order Laplace/1 -> Switch3/1
  Random Number1/1 -> Gain1/1
  Mux1/1 -> To Workspace1/1
  Sum1/1 -> Mux1/4, Saturation1/1
  Switch3/1 -> Mux1/2, Sum1/1

== system KTB1_SMAH/Sensor model 4 ==
  In1 : Inport
  Constant1 : Constant  Value=usenoise_XXXX
  Constant3 : Constant  Value=useideal_XXXX
  Constant4 : Constant  Value=use2ndFcn_XXXX
  Gain1 : Gain  Gain=max_XXXX*std_XXXX  SaturateOnIntegerOverflow=on  OutDataTypeStr=Inherit: Same as input  ParamDataTypeStr=Inherit: Same as input
  Mux1 : Mux  Inputs=5
  Product1 : Product  InputSameDT=on  SaturateOnIntegerOverflow=on  OutDataTypeStr=Inherit: Same as first input
  Random Number1 : RandomNumber  Variance=0.025  Seed=noiseseed_XXXX  SampleTime=1/2
  Saturation1 : Saturate  UpperLimit=max_XXXX  LowerLimit=min_XXXX
  Sum1 : Sum  Inputs=|++  InputSameDT=on  SaturateOnIntegerOverflow=on  OutDataTypeStr=Inherit: Same as first input
  Switch2 : Switch  Threshold=0.5
  Switch3 : Switch  Threshold=0.5
  To Workspace1 : ToWorkspace  VariableName=XXXXsensor  SampleTime=-1
  eight order Laplace : TransferFcn  Denominator=[ T_XXXX_8*T_XXXX_8*T_XXXX_8*T_XXXX_8*T_XXXX_8*T_XXXX_8*T_XXXX_8*T_XXXX_8, 8*T_XXXX_8*T_XXXX_8*T_XXXX_8*T_XXXX_8*T_XXXX_8*T_XXXX_8*T_XXXX_8, 28*T_XXXX_8*T_XXXX_8*T_XXXX_8*T_XXXX_8*T_XXXX_8*T_XXXX_8, 56*T_XXXX_8*T_XXXX_8*T_XXXX_8*T_XXXX_8*T_XXXX_8, 70*T_XXXX_8*T_XXXX_8*T_XXXX_8*T_XXXX_8, 56*T_XXXX_8*T_XXXX_8*T_XXXX_8, 28*T_XXXX_8*T_XXXX_8, 8* T_XXXX_8, 1]
  second order Laplace : TransferFcn  Denominator=[ T_XXXX_2*T_XXXX_2, 2*T_XXXX_2, 1]
  Out1 : Outport
  wires:
  Saturation1/1 -> Switch2/3
  In1/1 -> second order Laplace/1, Mux1/1, Switch2/1, eight order Laplace/1
  Constant1/1 -> Product1/1
  eight order Laplace/1 -> Switch3/3
  Constant4/1 -> Switch3/2
  Gain1/1 -> Product1/2
  Product1/1 -> Mux1/3, Sum1/2
  Switch2/1 -> Mux1/5, Out1/1
  Constant3/1 -> Switch2/2
  second order Laplace/1 -> Switch3/1
  Random Number1/1 -> Gain1/1
  Mux1/1 -> To Workspace1/1
  Sum1/1 -> Mux1/4, Saturation1/1
  Switch3/1 -> Mux1/2, Sum1/1

== system KTB1_SMAH/Sensor model 5 ==
  In1 : Inport
  Constant1 : Constant  Value=usenoise_XXXXX
  Constant3 : Constant  Value=useideal_XXXXX
  Constant4 : Constant  Value=use2ndFcn_XXXXX
  Gain1 : Gain  Gain=max_XXXXX*std_XXXXX  SaturateOnIntegerOverflow=on  OutDataTypeStr=Inherit: Same as input  ParamDataTypeStr=Inherit: Same as input
  Mux1 : Mux  Inputs=5
  Product1 : Product  InputSameDT=on  SaturateOnIntegerOverflow=on  OutDataTypeStr=Inherit: Same as first input
  Random Number1 : RandomNumber  Variance=0.025  Seed=noiseseed_XXXXX  SampleTime=1/2
  Saturation1 : Saturate  UpperLimit=max_XXXXX  LowerLimit=min_XXXXX
  Sum1 : Sum  Inputs=|++  InputSameDT=on  SaturateOnIntegerOverflow=on  OutDataTypeStr=Inherit: Same as first input
  Switch2 : Switch  Threshold=0.5
  Switch3 : Switch  Threshold=0.5
  To Workspace1 : ToWorkspace  VariableName=XXXXXsensor  SampleTime=-1
  eight order Laplace : TransferFcn  Denominator=[ T_XXXXX_8*T_XXXXX_8*T_XXXXX_8*T_XXXXX_8*T_XXXXX_8*T_XXXXX_8*T_XXXXX_8*T_XXXXX_8, 8*T_XXXXX_8*T_XXXXX_8*T_XXXXX_8*T_XXXXX_8*T_XXXXX_8*T_XXXXX_8*T_XXXXX_8, 28*T_XXXXX_8*T_XXXXX_8*T_XXXXX_8*T_XXXXX_8*T_XXXXX_8*T_XXXXX_8, 56*T_XXXXX_8*T_XXXXX_8*T_XXXXX_8*T_XXXXX_8*T_XXXXX_8, 70*T_XXXXX_8*T_XXXXX_8*T_XXXXX_8*T_XXXXX_8, 56*T_XXXXX_8*T_XXXXX_8*T_XXXXX_8, 28*T_XXXXX_8*T_XXXXX_8, 8* T_XXXXX_8, 1]
  second order Laplace : TransferFcn  Denominator=[ T_XXXXX_2*T_XXXXX_2, 2*T_XXXXX_2, 1]
  Out1 : Outport
  wires:
  Saturation1/1 -> Switch2/3
  In1/1 -> second order Laplace/1, Mux1/1, Switch2/1, eight order Laplace/1
  Constant1/1 -> Product1/1
  eight order Laplace/1 -> Switch3/3
  Constant4/1 -> Switch3/2
  Gain1/1 -> Product1/2
  Product1/1 -> Mux1/3, Sum1/2
  Switch2/1 -> Mux1/5, Out1/1
  Constant3/1 -> Switch2/2
  second order Laplace/1 -> Switch3/1
  Random Number1/1 -> Gain1/1
  Mux1/1 -> To Workspace1/1
  Sum1/1 -> Mux1/4, Saturation1/1
  Switch3/1 -> Mux1/2, Sum1/1

== system KTB1_SMAH/Discrete time P controller/1 ==
  In1 : Inport
  Injection time 1 : Step  Time=(5.1313509526065/20)*6  Before=1  After=0  SampleTime=0
  Product5 : Product
  To Workspace1 : ToWorkspace  VariableName=V_inj_1  SaveFormat=Timeseries  SampleTime=-1
  To Workspace6 : ToWorkspace  VariableName=t_inj_1  SaveFormat=Timeseries  SampleTime=-1
  Out1 : Outport  VectorParamsAs1DForOutWhenUnconnected=off
  wires:
  Product5/1 -> To Workspace1/1, Out1/1
  Injection time 1/1 -> Product5/1, To Workspace6/1
  In1/1 -> Product5/2

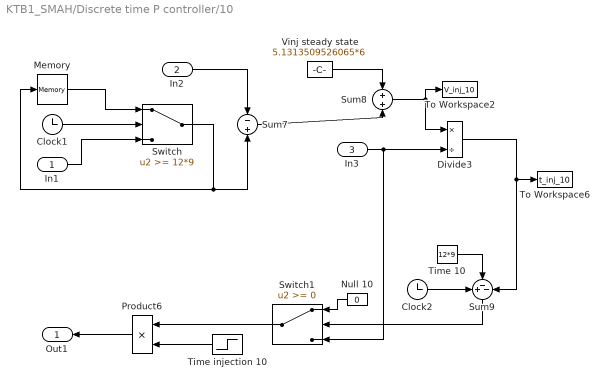
== system KTB1_SMAH/Discrete time P controller/10 ==
  In1 : Inport
  In2 : Inport  Port=2
  In3 : Inport  Port=3
  Clock1 : Clock
  Clock2 : Clock
  Divide3 : Product  Inputs=*/
  Memory : Memory
  Null 10 : Constant  Value=0
  Product6 : Product
  Sum7 : Sum  Inputs=-+
  Sum8 : Sum
  Sum9 : Sum  Inputs=+--
  Switch : Switch  Threshold=12*9
  Switch1 : Switch
  Time 10 : Constant  Value=12*9
  Time injection 10 : Step  Time=12*9  SampleTime=0
  To Workspace2 : ToWorkspace  VariableName=V_inj_10  SaveFormat=Timeseries  SampleTime=-1
  To Workspace6 : ToWorkspace  VariableName=t_inj_10  SaveFormat=Timeseries  SampleTime=-1
  Vinj steady state : Constant  Value=5.1313509526065*6
  Out1 : Outport  VectorParamsAs1DForOutWhenUnconnected=off
  wires:
  In1/1 -> Switch/3
  Time injection 10/1 -> Product6/2
  Switch/1 -> Memory/1, Sum7/2
  Time 10/1 -> Sum9/2
  Switch1/1 -> Product6/1
  Clock1/1 -> Switch/2
  Memory/1 -> Switch/1
  Null 10/1 -> Switch1/1
  Divide3/1 -> Sum9/3, To Workspace6/1
  Clock2/1 -> Sum9/1
  In2/1 -> Sum7/1
  Vinj steady state/1 -> Sum8/1
  In3/1 -> Switch1/3, Divide3/2
  Sum9/1 -> Switch1/2
  Sum7/1 -> Sum8/2
  Product6/1 -> Out1/1
  Sum8/1 -> Divide3/1, To Workspace2/1

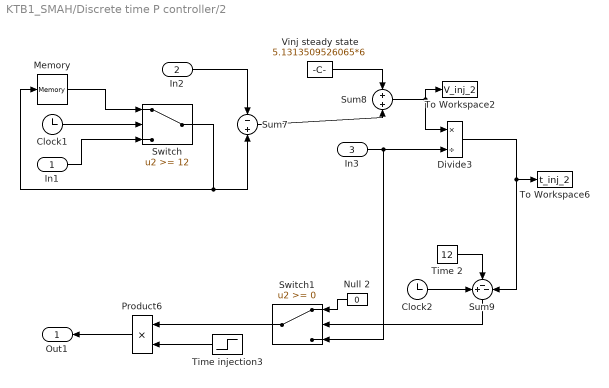
== system KTB1_SMAH/Discrete time P controller/2 ==
  In1 : Inport
  In2 : Inport  Port=2
  In3 : Inport  Port=3
  Clock1 : Clock
  Clock2 : Clock
  Divide3 : Product  Inputs=*/
  Memory : Memory
  Null 2 : Constant  Value=0
  Product6 : Product
  Sum7 : Sum  Inputs=-+
  Sum8 : Sum
  Sum9 : Sum  Inputs=+--
  Switch : Switch  Threshold=12
  Switch1 : Switch
  Time 2 : Constant  Value=12
  Time injection3 : Step  Time=12  SampleTime=0
  To Workspace2 : ToWorkspace  VariableName=V_inj_2  SaveFormat=Timeseries  SampleTime=-1
  To Workspace6 : ToWorkspace  VariableName=t_inj_2  SaveFormat=Timeseries  SampleTime=-1
  Vinj steady state : Constant  Value=5.1313509526065*6
  Out1 : Outport  VectorParamsAs1DForOutWhenUnconnected=off
  wires:
  In1/1 -> Switch/3
  Time injection3/1 -> Product6/2
  Switch/1 -> Memory/1, Sum7/2
  Time 2/1 -> Sum9/2
  Switch1/1 -> Product6/1
  Clock1/1 -> Switch/2
  Memory/1 -> Switch/1
  Null 2/1 -> Switch1/1
  Divide3/1 -> Sum9/3, To Workspace6/1
  Clock2/1 -> Sum9/1
  In2/1 -> Sum7/1
  Vinj steady state/1 -> Sum8/1
  In3/1 -> Switch1/3, Divide3/2
  Sum9/1 -> Switch1/2
  Sum7/1 -> Sum8/2
  Product6/1 -> Out1/1
  Sum8/1 -> Divide3/1, To Workspace2/1

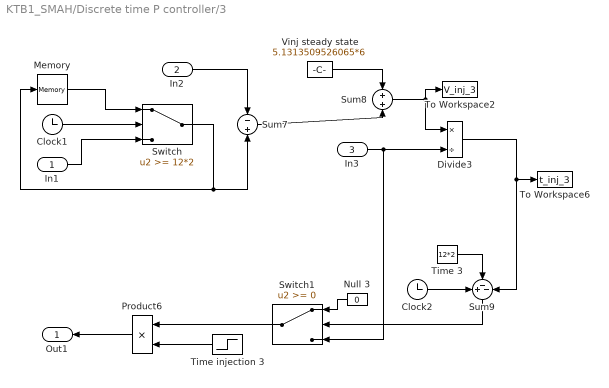
== system KTB1_SMAH/Discrete time P controller/3 ==
  In1 : Inport
  In2 : Inport  Port=2
  In3 : Inport  Port=3
  Clock1 : Clock
  Clock2 : Clock
  Divide3 : Product  Inputs=*/
  Memory : Memory
  Null 3 : Constant  Value=0
  Product6 : Product
  Sum7 : Sum  Inputs=-+
  Sum8 : Sum
  Sum9 : Sum  Inputs=+--
  Switch : Switch  Threshold=12*2
  Switch1 : Switch
  Time 3 : Constant  Value=12*2
  Time injection 3 : Step  Time=12*2  SampleTime=0
  To Workspace2 : ToWorkspace  VariableName=V_inj_3  SaveFormat=Timeseries  SampleTime=-1
  To Workspace6 : ToWorkspace  VariableName=t_inj_3  SaveFormat=Timeseries  SampleTime=-1
  Vinj steady state : Constant  Value=5.1313509526065*6
  Out1 : Outport  VectorParamsAs1DForOutWhenUnconnected=off
  wires:
  In1/1 -> Switch/3
  Time injection 3/1 -> Product6/2
  Switch/1 -> Memory/1, Sum7/2
  Time 3/1 -> Sum9/2
  Switch1/1 -> Product6/1
  Clock1/1 -> Switch/2
  Memory/1 -> Switch/1
  Null 3/1 -> Switch1/1
  Divide3/1 -> Sum9/3, To Workspace6/1
  Clock2/1 -> Sum9/1
  In2/1 -> Sum7/1
  Vinj steady state/1 -> Sum8/1
  In3/1 -> Switch1/3, Divide3/2
  Sum9/1 -> Switch1/2
  Sum7/1 -> Sum8/2
  Product6/1 -> Out1/1
  Sum8/1 -> Divide3/1, To Workspace2/1

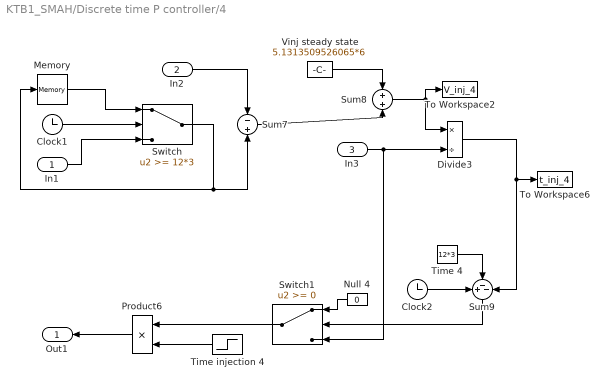
== system KTB1_SMAH/Discrete time P controller/4 ==
  In1 : Inport
  In2 : Inport  Port=2
  In3 : Inport  Port=3
  Clock1 : Clock
  Clock2 : Clock
  Divide3 : Product  Inputs=*/
  Memory : Memory
  Null 4 : Constant  Value=0
  Product6 : Product
  Sum7 : Sum  Inputs=-+
  Sum8 : Sum
  Sum9 : Sum  Inputs=+--
  Switch : Switch  Threshold=12*3
  Switch1 : Switch
  Time 4 : Constant  Value=12*3
  Time injection 4 : Step  Time=12*3  SampleTime=0
  To Workspace2 : ToWorkspace  VariableName=V_inj_4  SaveFormat=Timeseries  SampleTime=-1
  To Workspace6 : ToWorkspace  VariableName=t_inj_4  SaveFormat=Timeseries  SampleTime=-1
  Vinj steady state : Constant  Value=5.1313509526065*6
  Out1 : Outport  VectorParamsAs1DForOutWhenUnconnected=off
  wires:
  In1/1 -> Switch/3
  Time injection 4/1 -> Product6/2
  Switch/1 -> Memory/1, Sum7/2
  Time 4/1 -> Sum9/2
  Switch1/1 -> Product6/1
  Clock1/1 -> Switch/2
  Memory/1 -> Switch/1
  Null 4/1 -> Switch1/1
  Divide3/1 -> Sum9/3, To Workspace6/1
  Clock2/1 -> Sum9/1
  In2/1 -> Sum7/1
  Vinj steady state/1 -> Sum8/1
  In3/1 -> Switch1/3, Divide3/2
  Sum9/1 -> Switch1/2
  Sum7/1 -> Sum8/2
  Product6/1 -> Out1/1
  Sum8/1 -> Divide3/1, To Workspace2/1

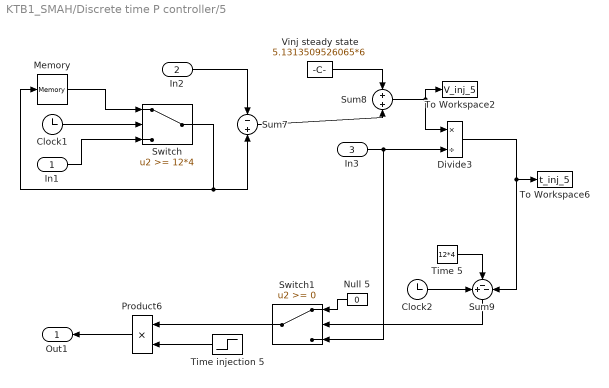
== system KTB1_SMAH/Discrete time P controller/5 ==
  In1 : Inport
  In2 : Inport  Port=2
  In3 : Inport  Port=3
  Clock1 : Clock
  Clock2 : Clock
  Divide3 : Product  Inputs=*/
  Memory : Memory
  Null 5 : Constant  Value=0
  Product6 : Product
  Sum7 : Sum  Inputs=-+
  Sum8 : Sum
  Sum9 : Sum  Inputs=+--
  Switch : Switch  Threshold=12*4
  Switch1 : Switch
  Time 5 : Constant  Value=12*4
  Time injection 5 : Step  Time=12*4  SampleTime=0
  To Workspace2 : ToWorkspace  VariableName=V_inj_5  SaveFormat=Timeseries  SampleTime=-1
  To Workspace6 : ToWorkspace  VariableName=t_inj_5  SaveFormat=Timeseries  SampleTime=-1
  Vinj steady state : Constant  Value=5.1313509526065*6
  Out1 : Outport  VectorParamsAs1DForOutWhenUnconnected=off
  wires:
  In1/1 -> Switch/3
  Time injection 5/1 -> Product6/2
  Switch/1 -> Memory/1, Sum7/2
  Time 5/1 -> Sum9/2
  Switch1/1 -> Product6/1
  Clock1/1 -> Switch/2
  Memory/1 -> Switch/1
  Null 5/1 -> Switch1/1
  Divide3/1 -> Sum9/3, To Workspace6/1
  Clock2/1 -> Sum9/1
  In2/1 -> Sum7/1
  Vinj steady state/1 -> Sum8/1
  In3/1 -> Switch1/3, Divide3/2
  Sum9/1 -> Switch1/2
  Sum7/1 -> Sum8/2
  Product6/1 -> Out1/1
  Sum8/1 -> Divide3/1, To Workspace2/1

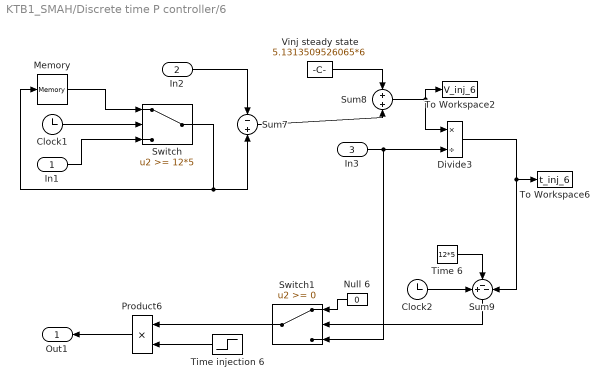
== system KTB1_SMAH/Discrete time P controller/6 ==
  In1 : Inport
  In2 : Inport  Port=2
  In3 : Inport  Port=3
  Clock1 : Clock
  Clock2 : Clock
  Divide3 : Product  Inputs=*/
  Memory : Memory
  Null 6 : Constant  Value=0
  Product6 : Product
  Sum7 : Sum  Inputs=-+
  Sum8 : Sum
  Sum9 : Sum  Inputs=+--
  Switch : Switch  Threshold=12*5
  Switch1 : Switch
  Time 6 : Constant  Value=12*5
  Time injection 6 : Step  Time=12*5  SampleTime=0
  To Workspace2 : ToWorkspace  VariableName=V_inj_6  SaveFormat=Timeseries  SampleTime=-1
  To Workspace6 : ToWorkspace  VariableName=t_inj_6  SaveFormat=Timeseries  SampleTime=-1
  Vinj steady state : Constant  Value=5.1313509526065*6
  Out1 : Outport  VectorParamsAs1DForOutWhenUnconnected=off
  wires:
  In1/1 -> Switch/3
  Time injection 6/1 -> Product6/2
  Switch/1 -> Memory/1, Sum7/2
  Time 6/1 -> Sum9/2
  Switch1/1 -> Product6/1
  Clock1/1 -> Switch/2
  Memory/1 -> Switch/1
  Null 6/1 -> Switch1/1
  Divide3/1 -> Sum9/3, To Workspace6/1
  Clock2/1 -> Sum9/1
  In2/1 -> Sum7/1
  Vinj steady state/1 -> Sum8/1
  In3/1 -> Switch1/3, Divide3/2
  Sum9/1 -> Switch1/2
  Sum7/1 -> Sum8/2
  Product6/1 -> Out1/1
  Sum8/1 -> Divide3/1, To Workspace2/1

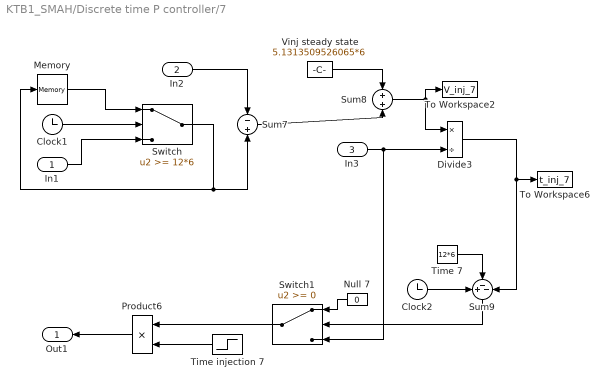
== system KTB1_SMAH/Discrete time P controller/7 ==
  In1 : Inport
  In2 : Inport  Port=2
  In3 : Inport  Port=3
  Clock1 : Clock
  Clock2 : Clock
  Divide3 : Product  Inputs=*/
  Memory : Memory
  Null 7 : Constant  Value=0
  Product6 : Product
  Sum7 : Sum  Inputs=-+
  Sum8 : Sum
  Sum9 : Sum  Inputs=+--
  Switch : Switch  Threshold=12*6
  Switch1 : Switch
  Time 7 : Constant  Value=12*6
  Time injection 7 : Step  Time=12*6  SampleTime=0
  To Workspace2 : ToWorkspace  VariableName=V_inj_7  SaveFormat=Timeseries  SampleTime=-1
  To Workspace6 : ToWorkspace  VariableName=t_inj_7  SaveFormat=Timeseries  SampleTime=-1
  Vinj steady state : Constant  Value=5.1313509526065*6
  Out1 : Outport  VectorParamsAs1DForOutWhenUnconnected=off
  wires:
  In1/1 -> Switch/3
  Time injection 7/1 -> Product6/2
  Switch/1 -> Memory/1, Sum7/2
  Time 7/1 -> Sum9/2
  Switch1/1 -> Product6/1
  Clock1/1 -> Switch/2
  Memory/1 -> Switch/1
  Null 7/1 -> Switch1/1
  Divide3/1 -> Sum9/3, To Workspace6/1
  Clock2/1 -> Sum9/1
  In2/1 -> Sum7/1
  Vinj steady state/1 -> Sum8/1
  In3/1 -> Switch1/3, Divide3/2
  Sum9/1 -> Switch1/2
  Sum7/1 -> Sum8/2
  Product6/1 -> Out1/1
  Sum8/1 -> Divide3/1, To Workspace2/1

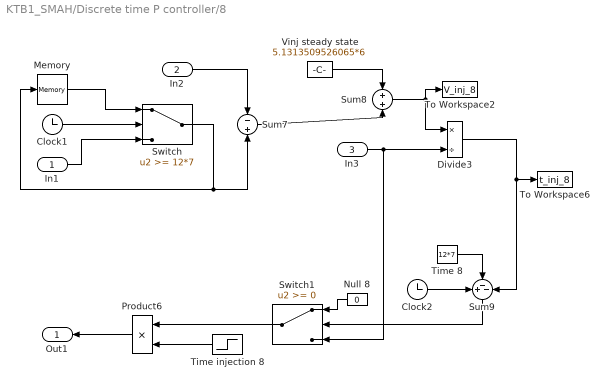
== system KTB1_SMAH/Discrete time P controller/8 ==
  In1 : Inport
  In2 : Inport  Port=2
  In3 : Inport  Port=3
  Clock1 : Clock
  Clock2 : Clock
  Divide3 : Product  Inputs=*/
  Memory : Memory
  Null 8 : Constant  Value=0
  Product6 : Product
  Sum7 : Sum  Inputs=-+
  Sum8 : Sum
  Sum9 : Sum  Inputs=+--
  Switch : Switch  Threshold=12*7
  Switch1 : Switch
  Time 8 : Constant  Value=12*7
  Time injection 8 : Step  Time=12*7  SampleTime=0
  To Workspace2 : ToWorkspace  VariableName=V_inj_8  SaveFormat=Timeseries  SampleTime=-1
  To Workspace6 : ToWorkspace  VariableName=t_inj_8  SaveFormat=Timeseries  SampleTime=-1
  Vinj steady state : Constant  Value=5.1313509526065*6
  Out1 : Outport  VectorParamsAs1DForOutWhenUnconnected=off
  wires:
  In1/1 -> Switch/3
  Time injection 8/1 -> Product6/2
  Switch/1 -> Memory/1, Sum7/2
  Time 8/1 -> Sum9/2
  Switch1/1 -> Product6/1
  Clock1/1 -> Switch/2
  Memory/1 -> Switch/1
  Null 8/1 -> Switch1/1
  Divide3/1 -> Sum9/3, To Workspace6/1
  Clock2/1 -> Sum9/1
  In2/1 -> Sum7/1
  Vinj steady state/1 -> Sum8/1
  In3/1 -> Switch1/3, Divide3/2
  Sum9/1 -> Switch1/2
  Sum7/1 -> Sum8/2
  Product6/1 -> Out1/1
  Sum8/1 -> Divide3/1, To Workspace2/1
